simulink model "cruise_control_topm"  (R2024a)
settings: Solver=VariableStepAuto  StartTime=0.0  StopTime=80  RelTol=1e-3
settings Model: DataDictionary=cruise_control_topm.sldd  Creator=timoravensbergen  LastModifiedBy=timoravensbergen

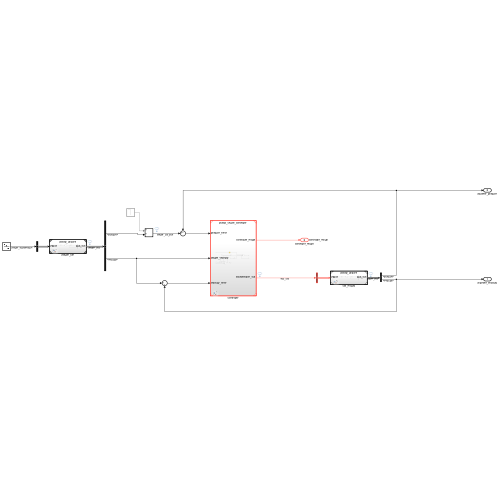
[thumbnail: Simulink's stored preview of the top-level diagram]
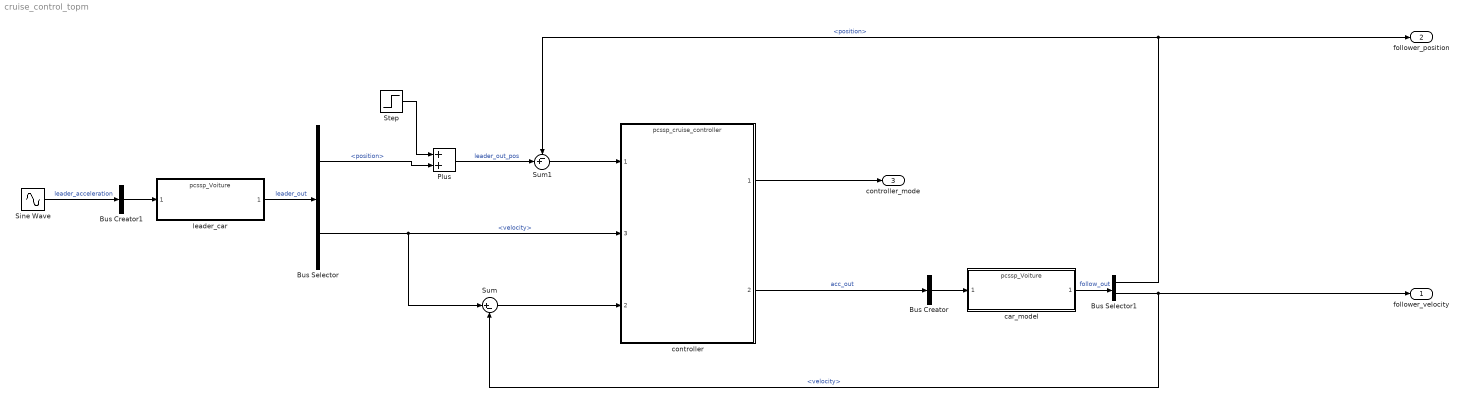
== system cruise_control_topm ==
  Bus Creator : BusCreator  Inputs=1  OutDataTypeStr=Bus: pcssp_voiture_inBus
      settings: InheritFromInputs=off
  Bus Creator1 : BusCreator  Inputs=1  OutDataTypeStr=Bus: pcssp_voiture_inBus
      settings: InheritFromInputs=off
  Bus Selector : BusSelector  OutputSignals=position,velocity
  Bus Selector1 : BusSelector  OutputSignals=position,velocity
  Plus : Sum
  Sine Wave : Sin  Amplitude=0.6  Frequency=0.2  SampleTime=0
  Step : Step  Time=15  After=-10  SampleTime=0
  Sum : Sum  Inputs=|+-
  Sum1 : Sum  Inputs=-+|
  car_model : ModelReference  ModelNameDialog=pcssp_Voiture.slx  SimulationMode=Normal  ModelReferenceVersion=1.5
  controller : ModelReference  ModelNameDialog=pcssp_cruise_controller.slx  SimulationMode=Normal  ModelReferenceVersion=1.25
      settings: PortSchema="{\"entries\":[{\"content\":{\"sides\":[{\"content\":{\"connectorIds\":[\"In1\",\"In3\",\"In2\"]},\"type\":\"ConnectorPlacement.EquallySpacedRectSide\",\"uuid\":\"15546cb6-b537-4f65-97b4-e561dd7dee88\"},{\"content\":{\"connectorIds\":[\"Out1\",\"Out2\"],\"side\":\"RIGHT\"},\"type\":\"ConnectorPlacement.EquallySpacedRectSide\",\"uuid\":\"ce9943e6-2727-45d3-b597-63f5aea8dcb6\"},{\"content\":{\"side\":\"TOP\"},\"type\":\"ConnectorPlacement.EquallySpacedRectSide\",\"uuid\":\"c11278aa-a31d-456e-9bfd-7e8f2a8e3a04\"}]},\"type\":\"ConnectorPlacement.EquallySpacedConnector\",\"uuid\":\"2d53bd98-e2fd-4ebb-8c06-ad9e770ad24a\"}],\"packageUris\":[\"http://schema.mathworks.com/mf0/Connector/R2020b\"],\"version\":\"1.0\"}"
  leader_car : ModelReference  ModelNameDialog=pcssp_Voiture.slx  SimulationMode=Normal  ModelReferenceVersion=1.5
  follower_velocity : Outport
  follower_position : Outport  Port=2
  controller_mode : Outport  Port=3  SignalName=controller_mode
  wires:
  leader_car/1 -> Bus Selector/1  "leader_out"
  Bus Selector1/1 -> Sum1/1, follower_position/1  "<position>"
  car_model/1 -> Bus Selector1/1  "follow_out"
  Sine Wave/1 -> Bus Creator1/1  "leader_acceleration"
  Bus Creator/1 -> car_model/1
  Bus Creator1/1 -> leader_car/1
  Bus Selector1/2 -> follower_velocity/1, Sum/2  "<velocity>"
  Bus Selector/2 -> Sum/1, controller/3  "<velocity>"
  Sum/1 -> controller/2
  Sum1/1 -> controller/1
  controller/1 -> controller_mode/1
  controller/2 -> Bus Creator/1  "acc_out"
  Step/1 -> Plus/1
  Bus Selector/1 -> Plus/2  "<position>"
  Plus/1 -> Sum1/2  "leader_out_pos"
